simulink model "model_of_system_gama"  (R2021a)
settings: Solver=VariableStepAuto  StartTime=0.0  StopTime=86400  RelTol=1e-3
libraries: fl_lib x49, nesl_utility x5, simulink x4
settings Model: OrderedModelArguments=off  Creator=SINA  LastModifiedBy=SINA
settings SolverCC: ZeroCrossAlgorithm=Adaptive
settings DebuggingCC: IgnoredZcDiagnostic=none

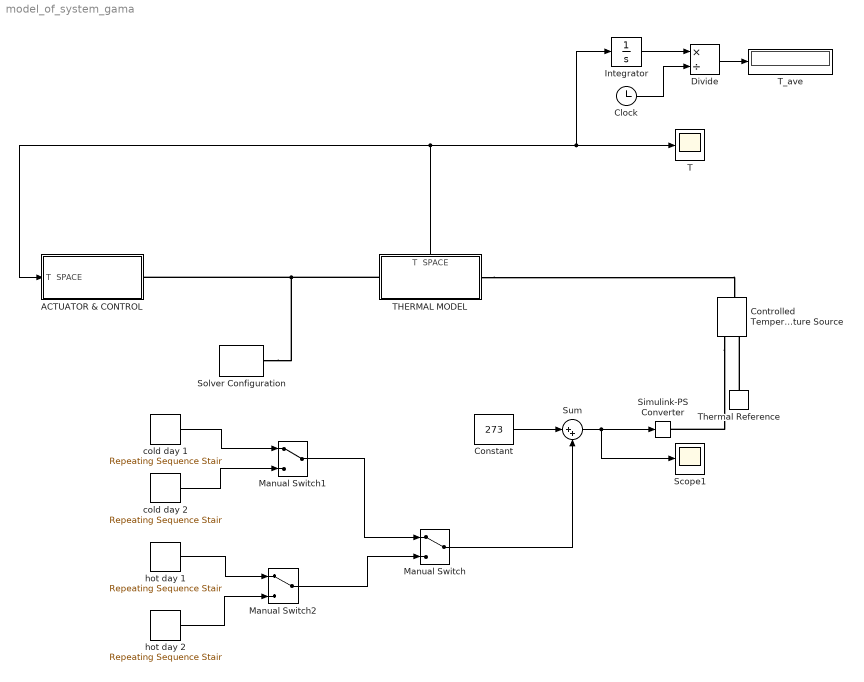
== system model_of_system_gama ==
  ACTUATOR & CONTROL : Subsystem
  Clock : Clock
  Constant : Constant  Value=273
  Controlled Temperature Source : fl_lib/Thermal/Thermal Sources/Controlled Temperature Source
  Divide : Product  Inputs=*/
  Integrator : Integrator
  Manual Switch : ManualSwitch
  Manual Switch1 : ManualSwitch
  Manual Switch2 : ManualSwitch
  Scope1 : Scope
  Simulink-PS Converter : nesl_utility/Simulink-PS Converter  PhysicalDomain=network_engine_domain  SubClassName=ps_input  LeftPortType=input  RightPortType=output  PseudoPeriodic=off  Frequencies=[]  NoiseDistribution=none  NoiseParameters=[]  Unit=K  AffineConversion=off  FilteringAndDerivatives=provide  SimscapeFilterOrder=1  InputFilterTimeConstant=0.001  UdotUserProvided=0
      settings: SourceProductBaseCode=PW,SS
  Solver Configuration : nesl_utility/Solver Configuration  PhysicalDomain=network_engine_domain  SubClassName=solver  LeftPortType=input  RightPortType=generic  Tones=[]  Harmonics=[]  SimulateNoise=off  Profile=off  UseLocalSampling=off  EnableSwitchedLinearOptims=on  FrequencyDomain=off  UseCCode=off  RelTol=0.001  AbsTol=1e-06  MinStep=1e-09  ToWorkspace=off  RevertToSquareIcSolve=off  NumHomotopyIterations=100  PhasorMode=off  PhasorModeNumHarmonics=1  DoDC=off  ResidualTolerance=1e-09  UseLocalSolver=off  LocalSolverChoice=NE_BACKWARD_EULER_ADVANCER  LocalSolverSampleTime=0.001  DoFixedCost=off  MaxNonlinIter=3  MaxModeIter=2  ComputeImpulses=off  ImpulseIterations=2  LinearAlgebra=auto  EquationFormulation=NE_TIME_EF  DelaysMemoryBudget=1024  AutomaticFiltering=on  FilteringTimeConstant=0.001  PartitionStorageMethod=AS_NEEDED  PartitionMemoryBudget=1024  PartitionMethod=ROBUST
      settings: SourceProductBaseCode=PW,SS
  Sum : Sum  Inputs=|++
  T : Scope
  "THERMAL MODEL " : Subsystem
      settings: PortSchema="{\"entries\":[{\"content\":{\"sides\":[{\"content\":{\"connectorIds\":[\"LConn1\"]},\"type\":\"ConnectorPlacement.EquallySpacedRectSide\",\"uuid\":\"d6720360-fd14-4102-8920-24b0f3e87daf\"},{\"content\":{\"connectorIds\":[\"RConn1\"],\"side\":\"RIGHT\"},\"type\":\"ConnectorPlacement.EquallySpacedRectSide\",\"uuid\":\"8de063fd-0e95-49b0-b131-452f09033aa1\"},{\"content\":{\"connectorIds\":[\"Out1\"],\"side\":\"TOP\"},\"type\":\"ConnectorPlacement.EquallySpacedRectSide\",\"uuid\":\"37599775-f873-4ff0-934d-fcf325c50c65\"}]},\"type\":\"ConnectorPlacement.EquallySpacedConnector\",\"uuid\":\"8fae0317-fc8f-430a-90e7-4ae7dd04f39d\"}],\"packageUris\":[\"http://schema.mathworks.com/mf0/Connector/R2020b\"],\"version\":\"1.0\"}"
  T_ave : Display
  Thermal Reference : fl_lib/Thermal/Thermal Elements/Thermal Reference
  "cold day 1 " : simulink/Sources/Repeating Sequence Stair  OutValues=|  tsamp=600  OutMin=[]  OutMax=[]  OutDataTypeStr=double  OutputDataTypeScalingMode=double  OutDataType=fixdt(0,8)  ConRadixGroup=Best Precision: Vector-wise  OutScaling=2^-12
      | [-0.50488
      | -0.18763
      | 0.17921
      | 0.35857
      | 0.10083
      | 0.09145
      | 0.21231
      | 0.21769
      | 0.50694
      | 0.75252
      | 0.77555
      | 0.77049
      | 0.7242
      | 0.62859
      | 0.50856
      | 0.16607
      | -0.55697
      | -0.74864
      | -0.78369
      | -0.77814
      | -0.57025
      | -0.5475
      | -0.64423
      | -0.70848
      | -0.7809
      | -0.80577
      | -0.99055
      | -1.1646
      | -1.253
      | -1.4825
      | -1.3655
      | -1.4522
      | -1.4623
      | -1.4657
      | -1.4438
      | -1.4408
      | -1.404
      | -1.3545
      | -1.1136
      | -0.98464
      | -0.69137
      | -0.25805
      | -0.14905
      | 0.06901
      | 0.30358
      | 0.21364
      | 0.26498
      | 0.50476
      | 0.85337
      | 1.1061
      | 1.6554
      | 1.6907
      | 1.9229
      | 1.9766
      | 2.046
      | 2.4259
      | 2.4742
      | 2.5851
      | 2.5979
      | 2.9236
      | 2.9203
      | 3.1039
      | 3.4189
      | 3.4003
      | 3.5325
      | 3.3863
      | 3.4948
      | 3.0974
      | 3.2078
      | 3.3736
      | 3.5806
      | 3.6768
      | 3.7653
      | 3.7023
      | 3.7098
      | 3.6711
      | 3.6008
      | 3.499
      | 3.3436
      | 3.2535
      | 3.1868
      | 3.0147
      | 3.0178
      | 3.0809
      | 3.2035
      | 3.1644
      | 3.1477
      | 3.0123
      | 3.0536
      | 3.101
      | 2.9914
      | 3.1268
      | 3.0077
      | 3.0066
      | 3.2039
      | 3.222
      | 2.7623
      | 2.5869
      | 2.4591
      | 2.181
      | 2.0403
      | 1.7878
      | 1.502
      | 1.4079
      | 1.3296
      | 1.3031
      | 1.1318
      | 1.0228
      | 0.90599
      | 0.83125
      | 0.83491
      | 0.78689
      | 0.8308
      | 0.78425
      | 0.7082
      | 0.64972
      | 0.61195
      | 0.60858
      | 0.52376
      | 0.4971
      | 0.41502
      | 0.34809
      | 0.28913
      | 0.13007
      | 0.09896
      | 0.13487
      | 0.03923
      | 0.01569
      | 0.05178
      | 0.14677
      | 0.17031
      | 0.12277
      | 0.11265
      | -0.01949
      | -0.04233
      | -0.10355
      | -0.14421
      | -0.17796
      | -0.13624
      | -0.10266
      | -0.10743
      | -0.15267
      | -0.23989
      | -0.32818
      | -0.3412
      | ]
  cold day 2 : simulink/Sources/Repeating Sequence Stair  OutValues=|  tsamp=600  OutMin=[]  OutMax=[]  OutDataTypeStr=double  OutputDataTypeScalingMode=double  OutDataType=fixdt(0,8)  ConRadixGroup=Best Precision: Vector-wise  OutScaling=2^-12
      | [-4.9
      | -4.9
      | -5
      | -4.9
      | -4.9
      | -4.8
      | -4.8
      | -4.8
      | -4.7
      | -4.7
      | -4.7
      | -4.7
      | -4.8
      | -4.8
      | -4.9
      | -4.9
      | -5
      | -5
      | -5
      | -5.1
      | -5.2
      | -5.2
      | -5.2
      | -5.2
      | -5.2
      | -5.2
      | -5.1
      | -5.3
      | -5.3
      | -5.3
      | -5.3
      | -5.3
      | -5.3
      | -5.2
      | -5.1
      | -5.1
      | -5
      | -4.8
      | -4.7
      | -4.6
      | -4.5
      | -4.5
      | -4.4
      | -4.2
      | -4.2
      | -3.9
      | -3.8
      | -3.6
      | -3.7
      | -3.5
      | -3.3
      | -3
      | -3
      | -2.7
      | -2.5
      | -2.5
      | -2.5
      | -2.5
      | -2.6
      | -2.5
      | -2.4
      | -2.4
      | -2.4
      | -2.3
      | -2.2
      | -2.3
      | -2.3
      | -2.2
      | -2.1
      | -2.1
      | -2
      | -1.9
      | -2
      | -1.9
      | -2
      | -2
      | -2
      | -2
      | -2
      | -2
      | -1.9
      | -2
      | -2
      | -2
      | -2
      | -2
      | -2
      | -2
      | -2
      | -1.9
      | -1.9
      | -1.8
      | -1.8
      | -1.8
      | -1.8
      | -1.9
      | -1.9
      | -1.8
      | -1.8
      | -1.8
      | -1.8
      | -1.8
      | -1.9
      | -1.9
      | -1.9
      | -2
      | -1.9
      | -1.9
      | -1.8
      | -1.9
      | -1.9
      | -2
      | -1.9
      | -1.9
      | -1.9
      | -1.9
      | -1.8
      | -1.8
      | -1.8
      | -1.8
      | -1.8
      | -1.8
      | -1.8
      | -1.8
      | -1.8
      | -1.8
      | -1.8
      | -1.8
      | -1.7
      | -1.8
      | -1.8
      | -1.8
      | -1.8
      | -1.7
      | -1.7
      | -1.8
      | -1.8
      | -1.8
      | -1.8
      | -1.8
      | -1.8
      | -1.9
      | -1.9
      | -1.9
      | -1.9
      | ]
  hot day 1 : simulink/Sources/Repeating Sequence Stair  OutValues=|  tsamp=600  OutMin=[]  OutMax=[]  OutDataTypeStr=double  OutputDataTypeScalingMode=double  OutDataType=fixdt(0,8)  ConRadixGroup=Best Precision: Vector-wise  OutScaling=2^-12
      | [22.172
      | 22.434
      | 22.456
      | 22.524
      | 22.565
      | 22.585
      | 22.669
      | 21.968
      | 22.073
      | 21.355
      | 21.194
      | 21.251
      | 21.405
      | 21.566
      | 21.683
      | 21.799
      | 21.8
      | 21.944
      | 22.289
      | 22.62
      | 22.667
      | 22.358
      | 22.001
      | 22.254
      | 22.328
      | 22.358
      | 22.686
      | 23.075
      | 23.311
      | 23.634
      | 24.082
      | 24.293
      | 25.056
      | 26.092
      | 25.953
      | 26.066
      | 26.444
      | 26.672
      | 27.3
      | 27.89
      | 28.466
      | 28.682
      | 29.137
      | 29.059
      | 29.449
      | 30.091
      | 30.485
      | 30.711
      | 30.819
      | 31.167
      | 31.647
      | 31.543
      | 31.947
      | 32.288
      | 32.795
      | 33.427
      | 33.474
      | 34.062
      | 33.947
      | 34.039
      | 34.088
      | 34.12
      | 34.123
      | 34.419
      | 34.506
      | 34.803
      | 34.94
      | 34.712
      | 35.015
      | 34.982
      | 34.973
      | 34.909
      | 35.148
      | 35.046
      | 35.129
      | 35.163
      | 35.11
      | 34.921
      | 35.012
      | 34.961
      | 34.947
      | 34.855
      | 34.669
      | 34.43
      | 34.583
      | 34.525
      | 34.233
      | 33.978
      | 33.947
      | 33.967
      | 33.715
      | 33.425
      | 33.251
      | 32.698
      | 32.287
      | 32.329
      | 31.934
      | 31.799
      | 31.425
      | 31.302
      | 31.088
      | 30.945
      | 30.43
      | 28.378
      | 26.349
      | 25.798
      | 25.296
      | 24.868
      | 24.665
      | 24.099
      | 23.808
      | 23.48
      | 23.341
      | 23.098
      | 22.645
      | 22.458
      | 22.436
      | 22.25
      | 22.01
      | 21.94
      | 21.951
      | 21.914
      | 21.856
      | 21.712
      | 21.646
      | 21.453
      | 21.266
      | 21.036
      | 20.949
      | 20.81
      | 20.588
      | 20.572
      | 20.619
      | 20.686
      | 20.628
      | 20.562
      | 20.413
      | 20.319
      | 20.407
      | 20.495
      | 20.493
      | 20.438
      | 20.212
      | 20.108
      | 19.915
      | ]
  hot day 2 : simulink/Sources/Repeating Sequence Stair  OutValues=|  tsamp=600  OutMin=[]  OutMax=[]  OutDataTypeStr=double  OutputDataTypeScalingMode=double  OutDataType=fixdt(0,8)  ConRadixGroup=Best Precision: Vector-wise  OutScaling=2^-12
      | [19.7
      | 19.8
      | 19.9
      | 19.6
      | 19.3
      | 19
      | 18.9
      | 18.8
      | 18.7
      | 18.6
      | 18.4
      | 18.3
      | 18.4
      | 18.5
      | 18.6
      | 18.6
      | 18.7
      | 18.5
      | 18.5
      | 18.5
      | 18.7
      | 18.9
      | 19.1
      | 19.6
      | 20
      | 20.3
      | 20.7
      | 20.9
      | 20.8
      | 20.7
      | 20.8
      | 21.4
      | 22.1
      | 22.7
      | 23
      | 23.7
      | 24.3
      | 25.2
      | 25.8
      | 25.8
      | 26.2
      | 26.5
      | 26.7
      | 26.7
      | 26.7
      | 27.8
      | 28.2
      | 28.4
      | 29.1
      | 29.5
      | 30.2
      | 30.8
      | 30.8
      | 31.2
      | 31.5
      | 31.4
      | 31.3
      | 31.3
      | 31.2
      | 31.4
      | 31.5
      | 31.5
      | 31.6
      | 31.5
      | 31.6
      | 31.3
      | 31.2
      | 31.2
      | 31.2
      | 31.9
      | 31.7
      | 31.4
      | 31.3
      | 31.6
      | 32.4
      | 32.3
      | 31.9
      | 32
      | 32.1
      | 32.1
      | 32.2
      | 32
      | 32.1
      | 32.1
      | 32.3
      | 32.3
      | 31.9
      | 31.4
      | 31.5
      | 31.5
      | 31
      | 30.6
      | 29.7
      | 28.9
      | 28.4
      | 28.1
      | 27.4
      | 26.6
      | 25.6
      | 24.5
      | 23.7
      | 22.9
      | 22.5
      | 22.2
      | 22
      | 21.9
      | 21.7
      | 21.4
      | 21.2
      | 21.1
      | 20.9
      | 20.9
      | 20.8
      | 20.7
      | 20.6
      | 20.2
      | 20
      | 19.9
      | 19.9
      | 19.9
      | 19.8
      | 19.6
      | 19.4
      | 19.1
      | 19
      | 19
      | 19
      | 18.9
      | 18.8
      | 18.7
      | 18.7
      | 18.3
      | 18
      | 17.7
      | 17.5
      | 17.5
      | 17.4
      | 17.3
      | 17.1
      | 17
      | 16.9
      | 16.8
      | 16.6
      | 16.5
      | 16.5
      | ]
  wires:
  "THERMAL MODEL "/1(T  SPACE) -> Integrator/1, T/1, ACTUATOR & CONTROL/1(T  SPACE)
  Constant/1 -> Sum/1
  Integrator/1 -> Divide/1
  Clock/1 -> Divide/2
  Divide/1 -> T_ave/1
  cold day 2/1 -> Manual Switch1/2
  "cold day 1 "/1 -> Manual Switch1/1
  Manual Switch1/1 -> Manual Switch/1
  hot day 1/1 -> Manual Switch2/1
  hot day 2/1 -> Manual Switch2/2
  Manual Switch2/1 -> Manual Switch/2
  Sum/1 -> Simulink-PS Converter/1, Scope1/1
  Manual Switch/1 -> Sum/2
  connections:
  Solver Configuration/RConn1 -- "THERMAL MODEL "/LConn1 -- ACTUATOR & CONTROL/RConn1
  Thermal Reference/LConn1 -- Controlled Temperature Source/RConn2
  Controlled Temperature Source/RConn1 -- Simulink-PS Converter/RConn1
  "THERMAL MODEL "/RConn1 -- Controlled Temperature Source/LConn1

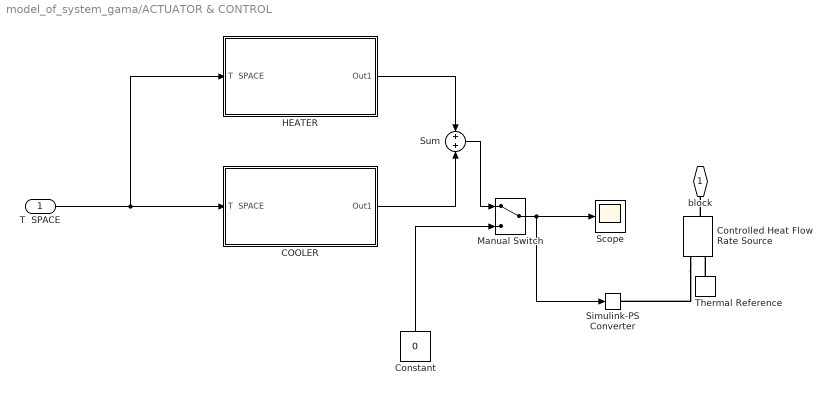
== system model_of_system_gama/ACTUATOR & CONTROL ==
  T  SPACE : Inport  SampleTime=1000
  COOLER : Subsystem
  Constant : Constant  Value=0
  Controlled Heat Flow Rate Source : fl_lib/Thermal/Thermal Sources/Controlled Heat Flow Rate Source
  HEATER : Subsystem
  Manual Switch : ManualSwitch
  Scope : Scope
  Simulink-PS Converter : nesl_utility/Simulink-PS Converter  PhysicalDomain=network_engine_domain  SubClassName=ps_input  LeftPortType=input  RightPortType=output  PseudoPeriodic=off  Frequencies=[]  NoiseDistribution=none  NoiseParameters=[]  Unit=J/s  AffineConversion=off  FilteringAndDerivatives=provide  SimscapeFilterOrder=1  InputFilterTimeConstant=0.001  UdotUserProvided=0
      settings: SourceProductBaseCode=PW,SS
  Sum : Sum
  Thermal Reference : fl_lib/Thermal/Thermal Elements/Thermal Reference
  " block" : PMIOPort  Side=Right
  wires:
  Manual Switch/1 -> Simulink-PS Converter/1, Scope/1
  Constant/1 -> Manual Switch/2
  T  SPACE/1 -> COOLER/1(T  SPACE), HEATER/1(T  SPACE)
  Sum/1 -> Manual Switch/1
  HEATER/1(Out1) -> Sum/1
  COOLER/1(Out1) -> Sum/2
  connections:
  Thermal Reference/LConn1 -- Controlled Heat Flow Rate Source/RConn2
  Controlled Heat Flow Rate Source/LConn1 -- " block"/RConn1
  Controlled Heat Flow Rate Source/RConn1 -- Simulink-PS Converter/RConn1

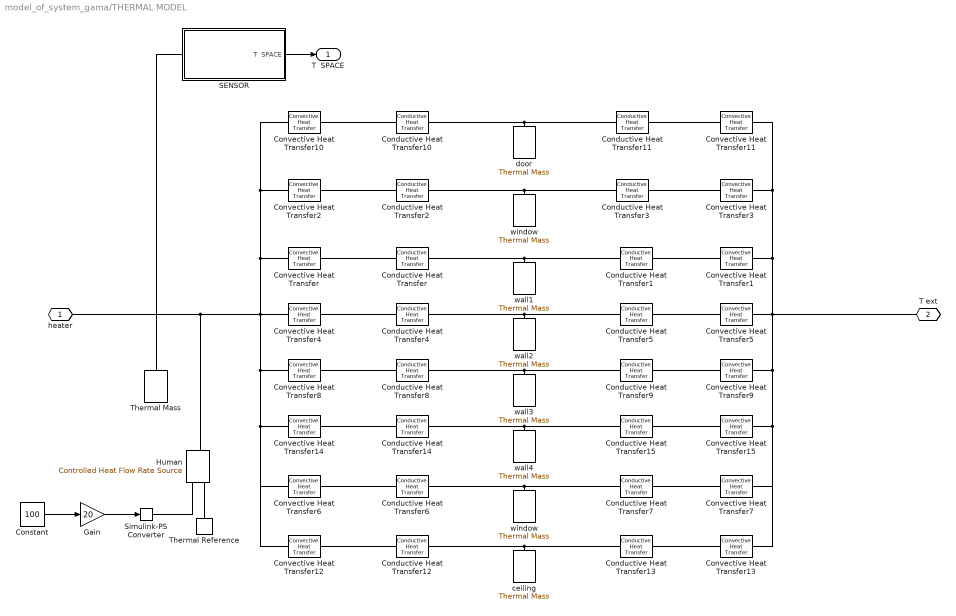
== system model_of_system_gama/THERMAL MODEL  ==
  " ceiling" : fl_lib/Thermal/Thermal Elements/Thermal Mass  mass=6400 kg  sp_heat=835 J/kg/K  T_specify=on  T_priority=None  T=295 K  T_nominal_specify=off  T_nominal_unit=K  T_nominal_value=1  Q_specify=off  Q_priority=None  Q=0 W  Q_nominal_specify=off  Q_nominal_unit=W  Q_nominal_value=1
  " window" : fl_lib/Thermal/Thermal Elements/Thermal Mass  mass=162 kg  sp_heat=840 J/kg/K  T_specify=on  T_priority=None  T=295 K  T_nominal_specify=off  T_nominal_unit=K  T_nominal_value=1  Q_specify=off  Q_priority=None  Q=0 W  Q_nominal_specify=off  Q_nominal_unit=W  Q_nominal_value=1
  Conductive Heat Transfer{,1,4..5} (4 alike) : fl_lib/Thermal/Thermal Elements/Conductive Heat Transfer  area=320 m^2  thickness=.2 m  th_cond=.038 W/(m*K)  T_specify=off  T_priority=None  T=0 K  T_nominal_specify=off  T_nominal_unit=K  T_nominal_value=1  Q_specify=off  Q_priority=None  Q=0 W  Q_nominal_specify=off  Q_nominal_unit=W  Q_nominal_value=1
  Conductive Heat Transfer10 : fl_lib/Thermal/Thermal Elements/Conductive Heat Transfer  area=7 m^2  thickness=0.04 m  th_cond=.78 W/(m*K)  T_specify=off  T_priority=None  T=0 K  T_nominal_specify=off  T_nominal_unit=K  T_nominal_value=1  Q_specify=off  Q_priority=None  Q=0 W  Q_nominal_specify=off  Q_nominal_unit=W  Q_nominal_value=1
  Conductive Heat Transfer11 : fl_lib/Thermal/Thermal Elements/Conductive Heat Transfer  area=7 m^2  thickness=.04 m  th_cond=.78 W/(m*K)  T_specify=off  T_priority=None  T=0 K  T_nominal_specify=off  T_nominal_unit=K  T_nominal_value=1  Q_specify=off  Q_priority=None  Q=0 W  Q_nominal_specify=off  Q_nominal_unit=W  Q_nominal_value=1
  Conductive Heat Transfer12 : fl_lib/Thermal/Thermal Elements/Conductive Heat Transfer  area=1000 m^2  thickness=0.1 m  th_cond=.038 W/(m*K)  T_specify=off  T_priority=None  T=0 K  T_nominal_specify=off  T_nominal_unit=K  T_nominal_value=1  Q_specify=off  Q_priority=None  Q=0 W  Q_nominal_specify=off  Q_nominal_unit=W  Q_nominal_value=1
  Conductive Heat Transfer13 : fl_lib/Thermal/Thermal Elements/Conductive Heat Transfer  area=1e-4 m^2  thickness=0.1 m  th_cond=.038 W/(m*K)  T_specify=off  T_priority=None  T=0 K  T_nominal_specify=off  T_nominal_unit=K  T_nominal_value=1  Q_specify=off  Q_priority=None  Q=0 W  Q_nominal_specify=off  Q_nominal_unit=W  Q_nominal_value=1
  Conductive Heat Transfer{8..9,14..15} (4 alike) : fl_lib/Thermal/Thermal Elements/Conductive Heat Transfer  area=150 m^2  thickness=.2 m  th_cond=.038 W/(m*K)  T_specify=off  T_priority=None  T=0 K  T_nominal_specify=off  T_nominal_unit=K  T_nominal_value=1  Q_specify=off  Q_priority=None  Q=0 W  Q_nominal_specify=off  Q_nominal_unit=W  Q_nominal_value=1
  Conductive Heat Transfer{2..3,6..7} (4 alike) : fl_lib/Thermal/Thermal Elements/Conductive Heat Transfer  area=6 m^2  thickness=.01 m  th_cond=.78 W/(m*K)  T_specify=off  T_priority=None  T=0 K  T_nominal_specify=off  T_nominal_unit=K  T_nominal_value=1  Q_specify=off  Q_priority=None  Q=0 W  Q_nominal_specify=off  Q_nominal_unit=W  Q_nominal_value=1
  Constant : Constant  Value=100
  Convective Heat Transfer{,1,4..5} (4 alike) : fl_lib/Thermal/Thermal Elements/Convective Heat Transfer  area=320 m^2  heat_tr_coeff=24 W/(m^2 * K)  T_specify=off  T_priority=None  T=0 K  T_nominal_specify=off  T_nominal_unit=K  T_nominal_value=1  Q_specify=off  Q_priority=None  Q=0 W  Q_nominal_specify=off  Q_nominal_unit=W  Q_nominal_value=1
  Convective Heat Transfer10 : fl_lib/Thermal/Thermal Elements/Convective Heat Transfer  area=7 m^2  heat_tr_coeff=26 W/(m^2 * K)  T_specify=off  T_priority=None  T=0 K  T_nominal_specify=off  T_nominal_unit=K  T_nominal_value=1  Q_specify=off  Q_priority=None  Q=0 W  Q_nominal_specify=off  Q_nominal_unit=W  Q_nominal_value=1
  Convective Heat Transfer11 : fl_lib/Thermal/Thermal Elements/Convective Heat Transfer  area=7 m^2  heat_tr_coeff=26 W/(m^2 * K)  T_specify=off  T_priority=None  T=0 K  T_nominal_specify=off  T_nominal_unit=K  T_nominal_value=1  Q_specify=off  Q_priority=None  Q=0 W  Q_nominal_specify=off  Q_nominal_unit=W  Q_nominal_value=1
  Convective Heat Transfer12 : fl_lib/Thermal/Thermal Elements/Convective Heat Transfer  area=1000 m^2  heat_tr_coeff=12 W/(m^2 * K)  T_specify=off  T_priority=None  T=0 K  T_nominal_specify=off  T_nominal_unit=K  T_nominal_value=1  Q_specify=off  Q_priority=None  Q=0 W  Q_nominal_specify=off  Q_nominal_unit=W  Q_nominal_value=1
  Convective Heat Transfer13 : fl_lib/Thermal/Thermal Elements/Convective Heat Transfer  area=1000 m^2  heat_tr_coeff=12 W/(m^2 * K)  T_specify=off  T_priority=None  T=0 K  T_nominal_specify=off  T_nominal_unit=K  T_nominal_value=1  Q_specify=off  Q_priority=None  Q=0 W  Q_nominal_specify=off  Q_nominal_unit=W  Q_nominal_value=1
  Convective Heat Transfer{8..9,14..15} (4 alike) : fl_lib/Thermal/Thermal Elements/Convective Heat Transfer  area=150 m^2  heat_tr_coeff=24 W/(m^2 * K)  T_specify=off  T_priority=None  T=0 K  T_nominal_specify=off  T_nominal_unit=K  T_nominal_value=1  Q_specify=off  Q_priority=None  Q=0 W  Q_nominal_specify=off  Q_nominal_unit=W  Q_nominal_value=1
  Convective Heat Transfer{2..3,6..7} (4 alike) : fl_lib/Thermal/Thermal Elements/Convective Heat Transfer  area=6 m^2  heat_tr_coeff=25 W/(m^2 * K)  T_specify=off  T_priority=None  T=0 K  T_nominal_specify=off  T_nominal_unit=K  T_nominal_value=1  Q_specify=off  Q_priority=None  Q=0 W  Q_nominal_specify=off  Q_nominal_unit=W  Q_nominal_value=1
  Gain : Gain  Gain=20
  Human : fl_lib/Thermal/Thermal Sources/Controlled Heat Flow Rate Source
  SENSOR : Subsystem
  Simulink-PS Converter : nesl_utility/Simulink-PS Converter  PhysicalDomain=network_engine_domain  SubClassName=ps_input  LeftPortType=input  RightPortType=output  PseudoPeriodic=off  Frequencies=[]  NoiseDistribution=none  NoiseParameters=[]  Unit=J/s  AffineConversion=off  FilteringAndDerivatives=provide  SimscapeFilterOrder=1  InputFilterTimeConstant=0.001  UdotUserProvided=0
      settings: SourceProductBaseCode=PW,SS
  Thermal Mass : fl_lib/Thermal/Thermal Elements/Thermal Mass  mass=10200 kg  sp_heat=1 J/kg/K  T_specify=on  T_priority=High  T=295 K  T_nominal_specify=off  T_nominal_unit=K  T_nominal_value=1  Q_specify=off  Q_priority=None  Q=0 W  Q_nominal_specify=off  Q_nominal_unit=W  Q_nominal_value=1
  Thermal Reference : fl_lib/Thermal/Thermal Elements/Thermal Reference
  door : fl_lib/Thermal/Thermal Elements/Thermal Mass  mass=165 kg  sp_heat=840 J/kg/K  T_specify=on  T_priority=None  T=295 K  T_nominal_specify=off  T_nominal_unit=K  T_nominal_value=1  Q_specify=off  Q_priority=None  Q=0 W  Q_nominal_specify=off  Q_nominal_unit=W  Q_nominal_value=1
  wall1 : fl_lib/Thermal/Thermal Elements/Thermal Mass  mass=122880 kg  sp_heat=835 J/kg/K  T_specify=on  T_priority=None  T=295 K  T_nominal_specify=off  T_nominal_unit=K  T_nominal_value=1  Q_specify=off  Q_priority=None  Q=0 W  Q_nominal_specify=off  Q_nominal_unit=W  Q_nominal_value=1
  wall2 : fl_lib/Thermal/Thermal Elements/Thermal Mass  mass=122880 kg  sp_heat=835 J/kg/K  T_specify=on  T_priority=None  T=295 K  T_nominal_specify=off  T_nominal_unit=K  T_nominal_value=1  Q_specify=off  Q_priority=None  Q=0 W  Q_nominal_specify=off  Q_nominal_unit=W  Q_nominal_value=1
  wall3 : fl_lib/Thermal/Thermal Elements/Thermal Mass  mass=57600 kg  sp_heat=835 J/kg/K  T_specify=on  T_priority=None  T=295 K  T_nominal_specify=off  T_nominal_unit=K  T_nominal_value=1  Q_specify=off  Q_priority=None  Q=0 W  Q_nominal_specify=off  Q_nominal_unit=W  Q_nominal_value=1
  wall4 : fl_lib/Thermal/Thermal Elements/Thermal Mass  mass=57600 kg  sp_heat=835 J/kg/K  T_specify=on  T_priority=None  T=295 K  T_nominal_specify=off  T_nominal_unit=K  T_nominal_value=1  Q_specify=off  Q_priority=None  Q=0 W  Q_nominal_specify=off  Q_nominal_unit=W  Q_nominal_value=1
  window : fl_lib/Thermal/Thermal Elements/Thermal Mass  mass=162 kg  sp_heat=840 J/kg/K  T_specify=on  T_priority=None  T=295 K  T_nominal_specify=off  T_nominal_unit=K  T_nominal_value=1  Q_specify=off  Q_priority=None  Q=0 W  Q_nominal_specify=off  Q_nominal_unit=W  Q_nominal_value=1
  heater : PMIOPort  Side=Left
  T ext : PMIOPort  Port=2  Side=Right
  T  SPACE : Outport  SampleTime=1
  wires:
  SENSOR/1(T  SPACE) -> T  SPACE/1
  Constant/1 -> Gain/1
  Gain/1 -> Simulink-PS Converter/1
  connections:
  Convective Heat Transfer/RConn1 -- Conductive Heat Transfer/LConn1
  Conductive Heat Transfer/RConn1 -- Conductive Heat Transfer1/LConn1 -- wall1/LConn1
  Convective Heat Transfer1/LConn1 -- Conductive Heat Transfer1/RConn1
  Conductive Heat Transfer3/LConn1 -- Conductive Heat Transfer2/RConn1 -- window/LConn1
  Convective Heat Transfer2/RConn1 -- Conductive Heat Transfer2/LConn1
  Convective Heat Transfer3/LConn1 -- Conductive Heat Transfer3/RConn1
  Conductive Heat Transfer5/LConn1 -- Conductive Heat Transfer4/RConn1 -- wall2/LConn1
  Convective Heat Transfer4/RConn1 -- Conductive Heat Transfer4/LConn1
  Convective Heat Transfer5/LConn1 -- Conductive Heat Transfer5/RConn1
  Conductive Heat Transfer6/RConn1 -- Conductive Heat Transfer7/LConn1 -- " window"/LConn1
  Convective Heat Transfer7/LConn1 -- Conductive Heat Transfer7/RConn1
  Convective Heat Transfer6/RConn1 -- Conductive Heat Transfer6/LConn1
  Convective Heat Transfer2/LConn1 -- Convective Heat Transfer10/LConn1 -- SENSOR/LConn1 -- heater/RConn1 -- Thermal Mass/LConn1 -- Human/LConn1 -- Convective Heat Transfer14/LConn1 -- Convective Heat Transfer12/LConn1 -- Convective Heat Transfer6/LConn1 -- Convective Heat Transfer8/LConn1 -- Convective Heat Transfer4/LConn1 -- Convective Heat Transfer/LConn1
  Conductive Heat Transfer8/RConn1 -- Conductive Heat Transfer9/LConn1 -- wall3/LConn1
  Convective Heat Transfer9/LConn1 -- Conductive Heat Transfer9/RConn1
  Convective Heat Transfer8/RConn1 -- Conductive Heat Transfer8/LConn1
  Conductive Heat Transfer10/RConn1 -- Conductive Heat Transfer11/LConn1 -- door/LConn1
  Convective Heat Transfer11/LConn1 -- Conductive Heat Transfer11/RConn1
  Convective Heat Transfer10/RConn1 -- Conductive Heat Transfer10/LConn1
  Convective Heat Transfer11/RConn1 -- Convective Heat Transfer15/RConn1 -- Convective Heat Transfer13/RConn1 -- Convective Heat Transfer7/RConn1 -- Convective Heat Transfer9/RConn1 -- Convective Heat Transfer5/RConn1 -- T ext/RConn1 -- Convective Heat Transfer1/RConn1 -- Convective Heat Transfer3/RConn1
  Conductive Heat Transfer13/LConn1 -- " ceiling"/LConn1 -- Conductive Heat Transfer12/RConn1
  Convective Heat Transfer13/LConn1 -- Conductive Heat Transfer13/RConn1
  Convective Heat Transfer12/RConn1 -- Conductive Heat Transfer12/LConn1
  Conductive Heat Transfer14/RConn1 -- wall4/LConn1 -- Conductive Heat Transfer15/LConn1
  Convective Heat Transfer15/LConn1 -- Conductive Heat Transfer15/RConn1
  Convective Heat Transfer14/RConn1 -- Conductive Heat Transfer14/LConn1
  Thermal Reference/LConn1 -- Human/RConn2
  Human/RConn1 -- Simulink-PS Converter/RConn1

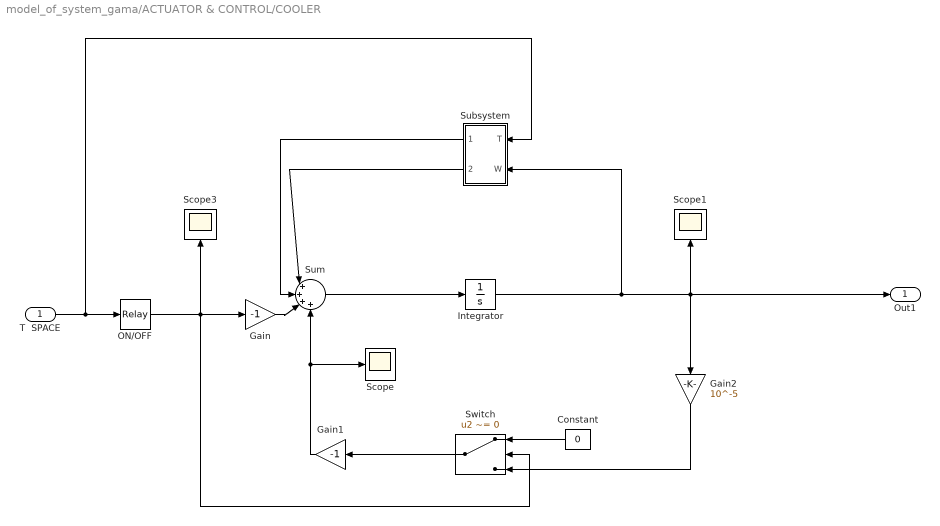
== system model_of_system_gama/ACTUATOR & CONTROL/COOLER ==
  T  SPACE : Inport
  Constant : Constant  Value=0
  Gain : Gain  Gain=-1
  Gain1 : Gain  Gain=-1
  Gain2 : Gain  Gain=10^-5
  Integrator : Integrator
  ON/OFF : Relay  OnSwitchValue=298  OffSwitchValue=295
  Scope : Scope
  Scope1 : Scope
  Scope3 : Scope
  Subsystem : Subsystem
  Sum : Sum  Inputs=|++++
  Switch : Switch  Criteria=u2 ~= 0
  Out1 : Outport
  wires:
  Subsystem/2(Out2) -> Sum/1
  Subsystem/1(Out1) -> Sum/2
  Gain/1 -> Sum/3
  Gain1/1 -> Scope/1, Sum/4
  T  SPACE/1 -> ON/OFF/1, Subsystem/1(T)
  ON/OFF/1 -> Switch/2, Gain/1, Scope3/1
  Integrator/1 -> Subsystem/2(W), Scope1/1, Gain2/1, Out1/1
  Sum/1 -> Integrator/1
  Switch/1 -> Gain1/1
  Constant/1 -> Switch/1
  Gain2/1 -> Switch/3

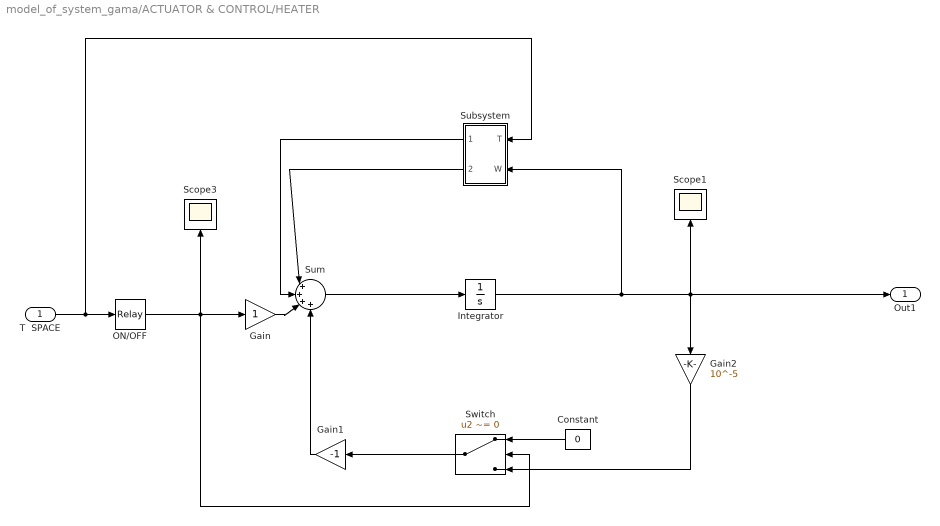
== system model_of_system_gama/ACTUATOR & CONTROL/HEATER ==
  T  SPACE : Inport
  Constant : Constant  Value=0
  Gain : Gain
  Gain1 : Gain  Gain=-1
  Gain2 : Gain  Gain=10^-5
  Integrator : Integrator
  ON/OFF : Relay  OnSwitchValue=293  OffSwitchValue=291  OnOutputValue=0  OffOutputValue=1
  Scope1 : Scope
  Scope3 : Scope
  Subsystem : Subsystem
  Sum : Sum  Inputs=|++++
  Switch : Switch  Criteria=u2 ~= 0
  Out1 : Outport
  wires:
  Constant/1 -> Switch/1
  Switch/1 -> Gain1/1
  Sum/1 -> Integrator/1
  Integrator/1 -> Out1/1, Gain2/1, Scope1/1, Subsystem/2(W)
  ON/OFF/1 -> Scope3/1, Gain/1, Switch/2
  T  SPACE/1 -> Subsystem/1(T), ON/OFF/1
  Gain1/1 -> Sum/4
  Gain/1 -> Sum/3
  Subsystem/1(Out1) -> Sum/2
  Subsystem/2(Out2) -> Sum/1
  Gain2/1 -> Switch/3

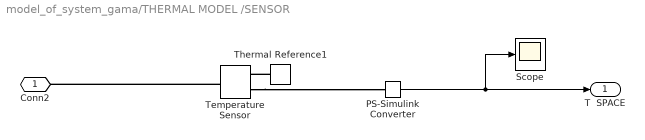
== system model_of_system_gama/THERMAL MODEL /SENSOR ==
  PS-Simulink Converter : nesl_utility/PS-Simulink Converter  PhysicalDomain=network_engine_domain  SubClassName=ps_output  LeftPortType=input  RightPortType=output  PseudoPeriodic=off  Frequencies=[]  Unit=K  AffineConversion=off
      settings: SourceProductBaseCode=PW,SS
  Scope : Scope
  Temperature Sensor : fl_lib/Thermal/Thermal Sensors/Temperature Sensor
  Thermal Reference1 : fl_lib/Thermal/Thermal Elements/Thermal Reference
  Conn2 : PMIOPort  Side=Left
  T  SPACE : Outport  SampleTime=1
  wires:
  PS-Simulink Converter/1 -> T  SPACE/1, Scope/1
  connections:
  Temperature Sensor/RConn2 -- PS-Simulink Converter/LConn1
  Temperature Sensor/LConn1 -- Conn2/RConn1
  Thermal Reference1/LConn1 -- Temperature Sensor/RConn1

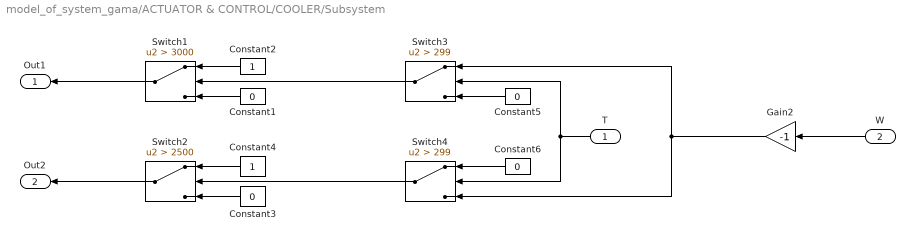
== system model_of_system_gama/ACTUATOR & CONTROL/COOLER/Subsystem ==
  T : Inport
  W : Inport  Port=2
  Constant{1,3,5..6} (4 alike) : Constant  Value=0
  Constant2 : Constant
  Constant4 : Constant
  Gain2 : Gain  Gain=-1
  Switch1 : Switch  Criteria=u2 > Threshold  Threshold=3000
  Switch2 : Switch  Criteria=u2 > Threshold  Threshold=2500
  Switch3 : Switch  Criteria=u2 > Threshold  Threshold=299
  Switch4 : Switch  Criteria=u2 > Threshold  Threshold=299
  Out1 : Outport
  Out2 : Outport  Port=2
  wires:
  Constant6/1 -> Switch4/1
  Switch4/1 -> Switch2/2
  Constant5/1 -> Switch3/3
  Switch2/1 -> Out2/1
  T/1 -> Switch4/2, Switch3/2
  Switch3/1 -> Switch1/2
  Switch1/1 -> Out1/1
  Constant1/1 -> Switch1/3
  Constant4/1 -> Switch2/1
  W/1 -> Gain2/1
  Constant2/1 -> Switch1/1
  Constant3/1 -> Switch2/3
  Gain2/1 -> Switch3/1, Switch4/3

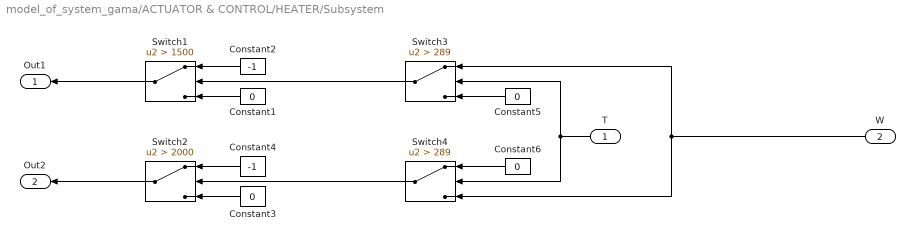
== system model_of_system_gama/ACTUATOR & CONTROL/HEATER/Subsystem ==
  T : Inport
  W : Inport  Port=2
  Constant{1,3,5..6} (4 alike) : Constant  Value=0
  Constant2 : Constant  Value=-1
  Constant4 : Constant  Value=-1
  Switch1 : Switch  Criteria=u2 > Threshold  Threshold=1500
  Switch2 : Switch  Criteria=u2 > Threshold  Threshold=2000
  Switch3 : Switch  Criteria=u2 > Threshold  Threshold=289
  Switch4 : Switch  Criteria=u2 > Threshold  Threshold=289
  Out1 : Outport
  Out2 : Outport  Port=2
  wires:
  Constant3/1 -> Switch2/3
  Constant2/1 -> Switch1/1
  W/1 -> Switch4/3, Switch3/1
  Constant4/1 -> Switch2/1
  Constant1/1 -> Switch1/3
  Switch1/1 -> Out1/1
  Switch3/1 -> Switch1/2
  T/1 -> Switch3/2, Switch4/2
  Switch2/1 -> Out2/1
  Constant5/1 -> Switch3/3
  Switch4/1 -> Switch2/2
  Constant6/1 -> Switch4/1
